simulink model "P1LVT"  (Simulink 6.0)
settings: Solver=ode45  StartTime=0.0  StopTime=10  RelTol=1e-3
settings Model: LastModifiedBy=Valdir Sampaio

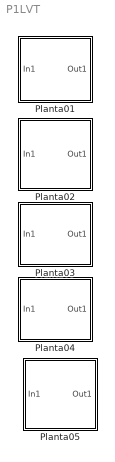
== system P1LVT ==
  Planta01 : Subsystem  mask{K1=1}
      mask prompts: K1 "Ganho"
      mask Display: disp('Planta P01')
  Planta02 : Subsystem  mask{K2=2}
      mask prompts: K2 "Ganho"
      mask Display: disp('Planta P02')
  Planta03 : Subsystem  mask{K3=0}
      mask prompts: K3 "Ganho"
      mask Display: disp('Planta P03')
  Planta04 : Subsystem  mask{K4=0}
      mask prompts: K4 "Ganho"
      mask Display: disp('Planta P04')
  Planta05 : Subsystem  mask{K5=1}
      mask prompts: K5 "Ganho"
      mask Display: disp('Planta P05')

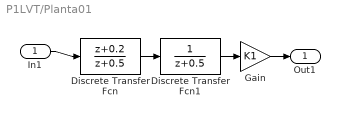
== system P1LVT/Planta01 ==
  In1 : Inport  Port=1  LatchInput=off
  Discrete Transfer Fcn : DiscreteTransferFcn  Numerator=[1 0.2]  SampleTime=0.25
  Discrete Transfer Fcn1 : DiscreteTransferFcn  SampleTime=0.25
  Gain : Gain  Gain=K1
  Out1 : Outport
  wires:
  Discrete Transfer Fcn/1 -> Discrete Transfer Fcn1/1
  Discrete Transfer Fcn1/1 -> Gain/1
  In1/1 -> Discrete Transfer Fcn/1
  Gain/1 -> Out1/1

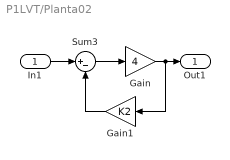
== system P1LVT/Planta02 ==
  In1 : Inport  Port=1  LatchInput=off
  Gain : Gain  Gain=4
  Gain1 : Gain  Orientation=left  Gain=K2
  Sum3 : Sum  Inputs=|+-
  Out1 : Outport
  wires:
  Sum3/1 -> Gain/1
  Gain1/1 -> Sum3/2
  Gain/1 -> Out1/1, Gain1/1
  In1/1 -> Sum3/1

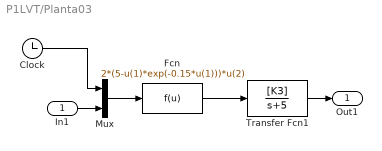
== system P1LVT/Planta03 ==
  In1 : Inport  Port=1  LatchInput=off
  Clock : Clock
      settings: Decimation=10
  Fcn : Fcn  Expr=2*(5-u(1)*exp(-0.15*u(1)))*u(2)
  Mux : Mux  Inputs=2
  Transfer Fcn1 : TransferFcn  Numerator=[K3]  Denominator=[1 5]
  Out1 : Outport
  wires:
  Clock/1 -> Mux/1
  Mux/1 -> Fcn/1
  Fcn/1 -> Transfer Fcn1/1
  Transfer Fcn1/1 -> Out1/1
  In1/1 -> Mux/2

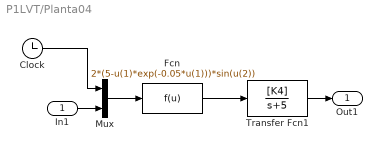
== system P1LVT/Planta04 ==
  In1 : Inport  Port=1  LatchInput=off
  Clock : Clock
      settings: Decimation=10
  Fcn : Fcn  Expr=2*(5-u(1)*exp(-0.05*u(1)))*sin(u(2))
  Mux : Mux  Inputs=2
  Transfer Fcn1 : TransferFcn  Numerator=[K4]  Denominator=[1 5]
  Out1 : Outport
  wires:
  Clock/1 -> Mux/1
  Mux/1 -> Fcn/1
  Fcn/1 -> Transfer Fcn1/1
  Transfer Fcn1/1 -> Out1/1
  In1/1 -> Mux/2

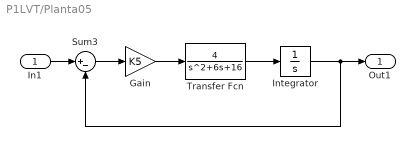
== system P1LVT/Planta05 ==
  In1 : Inport  Port=1  LatchInput=off
  Gain : Gain  Gain=K5
  Integrator : Integrator
  Sum3 : Sum  Inputs=|+-
  Transfer Fcn : TransferFcn  Numerator=[4]  Denominator=[1 6 16]
  Out1 : Outport
  wires:
  Sum3/1 -> Gain/1
  Gain/1 -> Transfer Fcn/1
  In1/1 -> Sum3/1
  Transfer Fcn/1 -> Integrator/1
  Integrator/1 -> Out1/1, Sum3/2
